simulink model "rotor_control_APPC"  (R2016a)
settings: Solver=VariableStepAuto  StartTime=0.0  StopTime=2  RelTol=1e-3
undefined symbols (not defined in the file or in its folder): load_amp, load_finish, load_start, measurement_variance, pulse_period, ref_amp, ref_mean, rotor_h, sinusoid_frequency
settings Model: Creator=Daniel  LastModifiedBy=mgreiff
settings DataIOCC: LimitDataPoints=on
settings DebuggingCC: AllowSymbolicDim=off
settings ModelReferenceCC: PropagateSignalLabelsOutOfModel=off
settings GRTTargetCC: GeneratePreprocessorConditionals=Use local settings

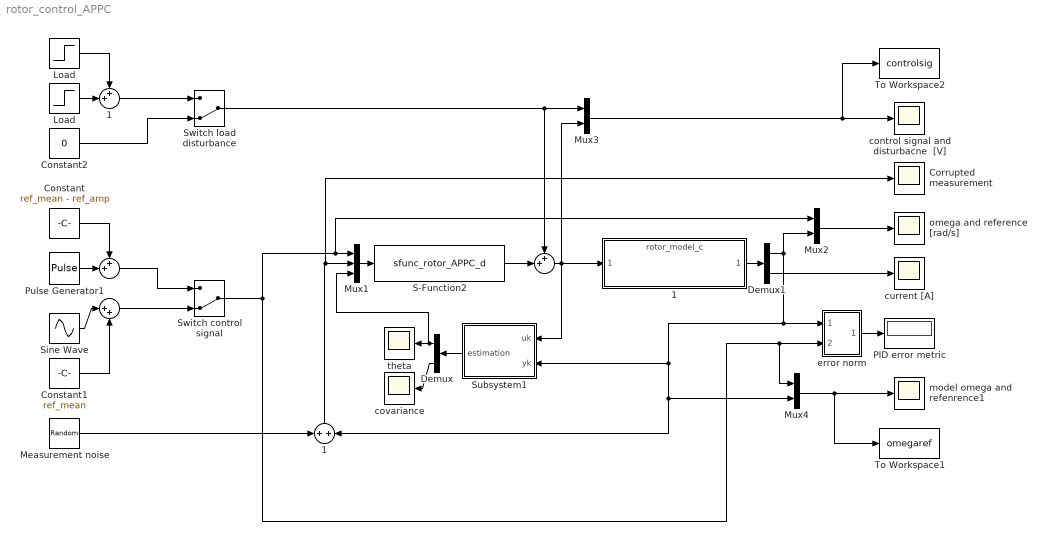
== system rotor_control_APPC ==
  " " : Sum  Inputs=++|
  "      " : Sum  Inputs=++|
  "       " : Sum  Inputs=|++
  "       1" : Sum
  "      1" : Sum  Inputs=++|
  "   1" : ModelReference  ModelNameDialog=rotor_model_c.slx  SimulationMode=Normal  ModelReferenceVersion=1.30
  " omega and reference [rad/s]" : Scope
  Constant : Constant  Value=ref_mean - ref_amp
  Constant1 : Constant  Value=ref_mean
  Constant2 : Constant  Value=0
  Corrupted measurement : Scope
  Demux : Demux  Outputs=[4,1]
  Demux1 : Demux  Outputs=2
  Load : Step  Time=load_finish  After=-load_amp  SampleTime=0
  "Load " : Step  Time=load_start  After=load_amp  SampleTime=0
  Measurement noise : RandomNumber  Variance=measurement_variance  SampleTime=rotor_h
  Mux1 : Mux  Inputs=3
  Mux2 : Mux  Inputs=2
  Mux3 : Mux  Inputs=2
  Mux4 : Mux  Inputs=2
  PID error metric : Display
  Pulse Generator1 : DiscretePulseGenerator  PulseType=Time based  Amplitude=ref_amp*2  Period=pulse_period  PulseWidth=50
  S-Function2 : S-Function  FunctionName=sfunc_rotor_APPC_d  Parameters=AMOPPCparam  SFunctionDeploymentMode=off  EnableBusSupport=off
  Sine Wave : Sin  Amplitude=200  Frequency=sinusoid_frequency  SampleTime=0
  Subsystem1 : Subsystem
  Switch control signal : ManualSwitch  CurrentSetting=0
  Switch load disturbance : ManualSwitch  CurrentSetting=0
  To Workspace1 : ToWorkspace  VariableName=omegaref  SaveFormat=Timeseries  SampleTime=-1
  To Workspace2 : ToWorkspace  VariableName=controlsig  SaveFormat=Timeseries  SampleTime=-1
  control signal and disturbacne  [V] : Scope
  covariance : Scope
  "current [A]   " : Scope
  error norm : Subsystem
  model omega and refenrence1 : Scope
  theta : Scope
  wires:
  Mux1/1 -> S-Function2/1
  Subsystem1/1(estimation) -> Demux/1
  Demux/1 -> Mux1/3, theta/1
  Demux/2 -> covariance/1
  "   1"/1 -> Demux1/1
  Constant/1 -> "      "/1
  Demux1/2 -> "current [A]   "/1
  "      "/1 -> Switch control signal/1
  Pulse Generator1/1 -> "      "/2
  Sine Wave/1 -> "       "/1
  "       "/1 -> Switch control signal/2
  Constant1/1 -> "       "/2
  " "/1 -> Subsystem1/1(uk), "   1"/1, Mux3/2
  Switch load disturbance/1 -> " "/1, Mux3/1
  Mux3/1 -> To Workspace2/1, control signal and disturbacne  [V]/1
  Switch control signal/1 -> Mux2/1, Mux1/1, error norm/2(In2), Mux4/1
  Mux4/1 -> model omega and refenrence1/1, To Workspace1/1
  "Load "/1 -> "      1"/1
  Load/1 -> "      1"/2
  error norm/1(Out1) -> PID error metric/1
  "      1"/1 -> Switch load disturbance/1
  Constant2/1 -> Switch load disturbance/2
  Demux1/1 -> "       1"/2, Mux4/2, Subsystem1/2(yk), error norm/1(In1), Mux2/2
  "       1"/1 -> Mux1/2, Corrupted measurement/1
  S-Function2/1 -> " "/2
  Mux2/1 -> " omega and reference [rad/s]"/1
  Measurement noise/1 -> "       1"/1

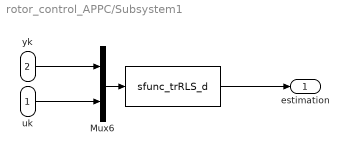
== system rotor_control_APPC/Subsystem1 ==
  uk : Inport
  yk : Inport  Port=2
  "   " : S-Function  FunctionName=sfunc_trRLS_d  Parameters=trRLSparam  SFunctionDeploymentMode=off  EnableBusSupport=off
  Mux6 : Mux  Inputs=2
  estimation : Outport
  wires:
  yk/1 -> Mux6/1
  uk/1 -> Mux6/2
  "   "/1 -> estimation/1
  Mux6/1 -> "   "/1

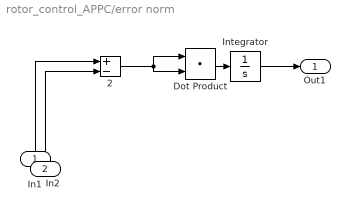
== system rotor_control_APPC/error norm ==
  In1 : Inport
  In2 : Inport  Port=2
  "      2" : Sum  Inputs=+-
  Dot Product : DotProduct  InputSameDT=on  OutDataTypeStr=Inherit: Inherit via internal rule
  Integrator : Integrator
  Out1 : Outport
  wires:
  "      2"/1 -> Dot Product/1, Dot Product/2
  Dot Product/1 -> Integrator/1
  In1/1 -> "      2"/1
  In2/1 -> "      2"/2
  Integrator/1 -> Out1/1
